simulink model "ads_test"  (Simulink 7.4)
settings: Solver=ode45  StartTime=0.0  StopTime=6000  RelTol=1e-3
values from neighbouring files (symbols this model uses):
  sensor_data = [1,3,[5000,1000,-3000],1,1,1,3.33,[0,0],1,1,0.2,[0.2,0.2,0.2],1,1]    [ads_test_sim.m]
  sim_par = [sat_par,init_JD,other_par]    [ads_test_sim.m]
libraries: aausat3_lib x7
settings Model: Creator=KF Jensen  LastModifiedBy=Administrator
settings DataIOCC: LimitDataPoints=off

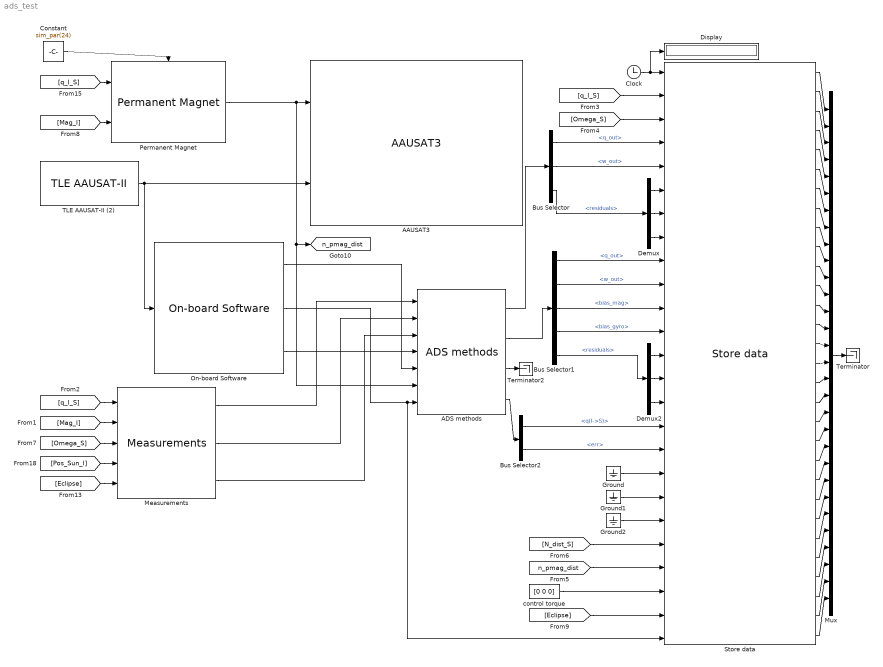
== system ads_test ==
  AAUSAT3 : aausat3_lib/AAUSAT3  SystemSampleTime=-1  r_com_s=sim_par(1:3)  sat_temp_start=293.15  mass_sc=sim_par(4)  Dim=[0.1,0.1,0.11]  inertia_c=sim_par(5:7)  init_jd=sim_par(19)  q_s_c=sim_par(8:11)  q_init_I_S=sim_par(12:15)  w_init_s=sim_par(16:18)  Cd=2  rho=5e-14  solar_m_flux=4.5565e-6  solar_absorb_coeff=1.5  theta_e=65  refldata=load('lib/AlbedoToolbox-1.0/refl_data/2005/ga050101-051231')  redfac=1  Ts=1  enable_sensor_emulation=on  enable_env_disturbance=on
  ADS methods : aausat3_lib/ADS/ADS methods  SystemSampleTime=-1  f_sample=sim_par(23)  svd_weigth=sim_par(25:27)  q0_guess=sim_par(12:15)  enable_ukf_simple=on  enable_ukf_bias=on  enable_ukf_bias_inertia=off  enable_svd=on
  Bus Selector : BusSelector  OutputSignals=signal1.q_out,signal1.w_out,signal1.residuals
  Bus Selector1 : BusSelector  OutputSignals=signal2.q_out,signal2.w_out,signal2.bias_mag,signal2.bias_gyro,signal2.residuals
  Bus Selector2 : BusSelector  OutputSignals=q(I->S),err
  Clock : Clock
  Constant : Constant  Value=sim_par(24)  OutDataType=fixdt(1, 16)  OutScaling=2^0
  Demux : Demux  Outputs=3
  Demux2 : Demux  Outputs=3
  Display : Display
  Ground : Ground
  Ground1 : Ground
  Ground2 : Ground
  Measurements : aausat3_lib/Sensor Emulation/Measurements  SystemSampleTime=-1  s_freq_mag=sensor_data(1)  noise_mag=sensor_data(2)  bias_mag=sensor_data(3:5)  heading_mag=sensor_data(6)  tilt_mag=sensor_data(7)  s_freq_sun=sensor_data(8)  noise_sun=sensor_data(9)  bias_sun=sensor_data(10:11)  nr_sample_sun=sensor_data(12)  s_freq_gyro=sensor_data(13)  noise_gyro=sensor_data(14)  bias_gyro=sensor_data(15:17)  heading_gyro=sensor_data(18)  tilt_gyro=sensor_data(19)
  Mux : Mux  Inputs=30
  On-board Software : aausat3_lib/On-board Software  SystemSampleTime=-1  init_jd=sim_par(20)  igrf_order=8  theta_e=65  f_sample=sim_par(22)
  Permanent Magnet : aausat3_lib/Actuator Emulation/Permanent Magnet  SystemSampleTime=-1  mag_moment=sim_par(27)
  Store data : aausat3_lib/Other Model Utilities/Store data  SystemSampleTime=-1  f_sample=sim_par(21)  enable_t=on  enable_att=on  enable_w=on  enable_att_ukf=on  enable_w_ukf=on  enable_r_sun=on  enable_r_mag=on  enable_r_w=on  enable_eia=on  enable_eiw=on  enable_att_ukf_bias=on  enable_w_ukf_bias=on  enable_b_mag=on  enable_b_gyro=on  enable_r_sun_ukf_bias=on  enable_r_mag_ukf_bias=on  enable_r_w_ukf_bias=on  enable_eia_ukf_bias=on  enable_eiw_ukf_bias=on  enable_att_svd=on  enable_svd_att_err=on  enable_svd_err=on  enable_tictoc=on  enable_tictoc_ukf_bias=on  enable_tictoc_svd=on  enable_n_dist=on  enable_n_pmag=on  enable_n_con=on  enable_eclip_sw=on  enable_eclip_real=on
  TLE AAUSAT-II (2) : aausat3_lib/Orbit and Ephemeris/TLE AAUSAT-II  SystemSampleTime=-1  satname='AAUSAT-II'  JulianDay=09321.69542252  xndt2o=0.00000555  xndd6o=0.0  bstar=.76898e-4  xincl=97.9251  xnodeo=24.1597  eo=0.0014245  omegao=254.1774  xmo=105.7862  xno=14.81823818  ts=1
  Terminator : Terminator
  Terminator2 : Terminator
  control torque : Constant  Value=[0 0 0]  OutDataType=fixdt(1, 16)  OutScaling=2^0
  tag scope: n_pmag_dist=global
  wires:
  Constant/1 -> Permanent Magnet/Enable
  [q_I_S] -> Permanent Magnet/1
  [Mag_I] -> Permanent Magnet/2
  Permanent Magnet/1 -> AAUSAT3/1, [n_pmag_dist], ADS methods/6
  TLE AAUSAT-II (2)/1 -> AAUSAT3/2, On-board Software/1
  [q_I_S] -> Measurements/1
  [Mag_I] -> Measurements/2
  [Omega_S] -> Measurements/3
  [Pos_Sun_I] -> Measurements/4
  [Eclipse] -> Measurements/5
  On-board Software/2 -> ADS methods/7, Store data/25
  Measurements/1 -> ADS methods/1
  Measurements/2 -> ADS methods/2
  Measurements/3 -> ADS methods/3
  On-board Software/3 -> ADS methods/4
  On-board Software/1 -> ADS methods/5
  ADS methods/1 -> Bus Selector/1
  ADS methods/2 -> Bus Selector1/1
  ADS methods/3 -> Terminator2/1
  Bus Selector/3 -> Demux/1  "<residuals>"
  Clock/1 -> Store data/1, Display/1
  [q_I_S] -> Store data/2
  [Omega_S] -> Store data/3
  Bus Selector/1 -> Store data/4  "<q_out>"
  Bus Selector/2 -> Store data/5  "<w_out>"
  Demux/1 -> Store data/6
  Demux/2 -> Store data/7
  Demux/3 -> Store data/8
  Demux2/1 -> Store data/13
  Demux2/2 -> Store data/14
  Demux2/3 -> Store data/15
  Bus Selector1/5 -> Demux2/1  "<residuals>"
  Bus Selector1/1 -> Store data/9  "<q_out>"
  Bus Selector1/2 -> Store data/10  "<w_out>"
  Bus Selector1/3 -> Store data/11  "<bias_mag>"
  Bus Selector1/4 -> Store data/12  "<bias_gyro>"
  Ground/1 -> Store data/18
  Ground1/1 -> Store data/19
  [N_dist_S] -> Store data/21
  [n_pmag_dist] -> Store data/22
  control torque/1 -> Store data/23
  [Eclipse] -> Store data/24
  Ground2/1 -> Store data/20
  ADS methods/4 -> Bus Selector2/1
  Bus Selector2/1 -> Store data/16  "<q(I->S)>"
  Mux/1 -> Terminator/1
  Bus Selector2/2 -> Store data/17  "<err>"
  Store data/1 -> Mux/1
  Store data/2 -> Mux/2
  Store data/3 -> Mux/3
  Store data/4 -> Mux/4
  Store data/5 -> Mux/5
  Store data/6 -> Mux/6
  Store data/7 -> Mux/7
  Store data/8 -> Mux/8
  Store data/9 -> Mux/9
  Store data/10 -> Mux/10
  Store data/11 -> Mux/11
  Store data/12 -> Mux/12
  Store data/13 -> Mux/13
  Store data/14 -> Mux/14
  Store data/15 -> Mux/15
  Store data/16 -> Mux/16
  Store data/17 -> Mux/17
  Store data/18 -> Mux/18
  Store data/19 -> Mux/19
  Store data/20 -> Mux/20
  Store data/21 -> Mux/21
  Store data/22 -> Mux/22
  Store data/23 -> Mux/23
  Store data/24 -> Mux/24
  Store data/25 -> Mux/25
  Store data/26 -> Mux/26
  Store data/27 -> Mux/27
  Store data/28 -> Mux/28
  Store data/29 -> Mux/29
  Store data/30 -> Mux/30
